simulink model "sysgenPatternGenerator"  (Simulink 7.1)
settings: Solver=VariableStepDiscrete  StartTime=0.0  StopTime=30000  RelTol=1e-3
PreLoadFcn:
  | load rgb;
  | fill_pattern_gen_program_store;
InitFcn:
  | load rgb;
  | fill_pattern_gen_program_store;
StopFcn:
  | makematrix(red, blue, green);
libraries: xbsIndex_r4 x47, xbsCopyrightNotice_r4 x1
settings Model: Creator=singhj  LastModifiedBy=sps
settings OptimizationCC: InlineInvariantSignals=on
settings DebuggingCC: SaveWithParameterizedLinksMsg=none  SignalResolutionControl=TryResolveAllWithWarning  SolverPrmCheckMsg=none  MultiTaskDSMMsg=warning  MultiTaskCondExecSysMsg=none  StrictBusMsg=None
settings RTWCC: IncludeERTFirstTime=on
settings GRTTargetCC: TargetFcnLib=ansi_tfl_tmw.mat

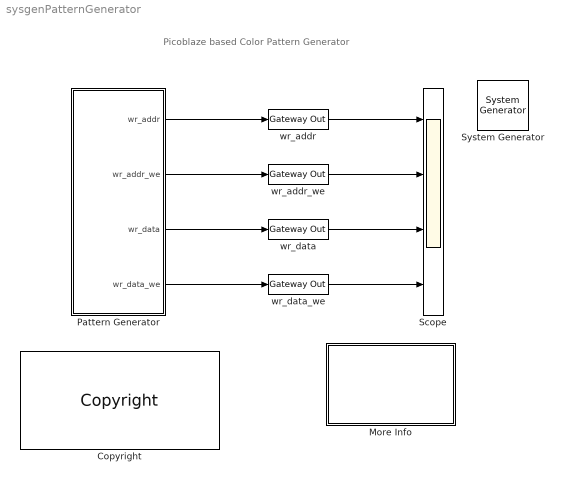
== system sysgenPatternGenerator ==
  note: Picoblaze based Color Pattern Generator
  " System Generator" : xbsIndex_r4/ System Generator  Tag=genX  SystemSampleTime=-1  xilinxfamily=virtex6  part=xc6vlx240t  speed=-1  package=ff1156  synthesis_tool=XST  clock_wrapper=Clock Enables  directory=./netlist  testbench=on  simulink_period=1  sysclk_period=10  dcm_input_clock_period=100  incr_netlist=off  trim_vbits=Everywhere in SubSystem  dbl_ovrd=According to Block Masks  core_generation=According to Block Masks  run_coregen=off  deprecated_control=off  eval_field=0  block_type=sysgen
      settings: block_version=9.2.00
  Copyright : xbsCopyrightNotice_r4/Copyright  copyrighttext="Copyright (c) 2010  by  Xilinx, Inc. All rights reserved.<br><br>This file contains proprietary, confidential information of Xilinx, Inc., is distributed under licensefrom Xilinx, Inc., and may be used, copied and/or disclosed only pursuant to the terms of a valid licenseagreement with Xilinx, Inc. Xilinx hereby grants you a license to use this file solely for design,simulation, implementation and creation of design files limited to Xilinx devices or technologies. Use with non-Xilinx devices or technologies is expressly prohibited and immediately terminates your license unless covered by a separate agreement.<br><br>Xilinx is providing this design, code, or information \"as-is\" solely for use in developing programs and solutions for Xilinx devices, with no obligation on the part of Xilinx to provide support. By providingthis design, code, or information as one possible implementation of this feature, application or standard,Xilinx is making no representation that this implementation is free from any claims of infringement. Youare responsible for obtaining any rights you may require for your implementation. Xilinx expressly disclaimsany warranty whatsoever with respect to the adequacy of the implementation, including but not limited to anywarranties or representations that this implementation is free from claims of infringement, implied warrantiesof merchantability or fitness for a particular purpose.<br><br>Xilinx products are not intended for use in life support appliances, devices, or systems. Use in such applications is expressly prohibited.<br><br>Any modifications that are made to the Source Code are done at the user's sole risk and will be unsupported.<br><br>This copyright and support notice must be retained as part of this text at all times. (c) Copyright 1995-2010 Xilinx, Inc. All rights reserved."  block_type=copyright
      settings: block_version=10.1.00
      settings: infoedit=|
      | Copyright(C) 2008 by  Xilinx, Inc. All rights reserved.<br>
      | <br>
      | This file contains proprietary, confidential information of Xilinx, Inc., is distributed under license
      | from Xilinx, Inc., and may be used, copied and/or disclosed only pursuant to the terms of a valid license
      | agreement with Xilinx, Inc. Xilinx hereby grants you a license to use this file solely for design,
      | simulation, implementation and creation of design files limited to Xilinx devices or technologies. Use
      | with non-Xilinx devices or technologies is expressly prohibited and immediately terminates your license
      | unless covered by a separate agreement.<br>
      | <br>
      | Xilinx is providing this design, code, or information "as-is" solely for use in developing programs and
      | solutions for Xilinx devices, with no obligation on the part of Xilinx to provide support. By providing
      | this design, code, or information as one possible implementation of this feature, application or standard,
      | Xilinx is making no representation that this implementation is free from any claims of infringement. You
      | are responsible for obtaining any rights you may require for your implementation. Xilinx expressly disclaims
      | any warranty whatsoever with respect to the adequacy of the implementation, including but not limited to any
      | warranties or representations that this implementation is free from claims of infringement, implied warranties
      | of merchantability or fitness for a particular purpose.<br>
      | <br>
      | Xilinx products are not intended for use in life support appliances, devices, or systems. Use in such
      | applications is expressly prohibited.<br>
      | <br>
      | Any modifications that are made to the Source Code are done at the user's sole risk and will be unsupported.<br>
      | <br>
      | This copyright and support notice must be retained as part of this text at all times.
      | (c) Copyright 1995-2008 Xilinx, Inc. All rights reserved.
  More Info : Subsystem
      mask Display: disp('Double click\n for\n more information.')
  Pattern Generator : Subsystem
  Scope : Scope  NumInputPorts=4
      settings: YMin=1.02005e+009~0~0~0  YMax=1.12743e+009~1~1.75e+007~1
  wr_addr : xbsIndex_r4/Gateway Out  hdl_port=on  timing_constraint=None  locs_specified=off  LOCs={}  block_type=gatewayout
      settings: infoedit="Gateway out block.  Converts Xilinx fixed point inputs into ouputs of type Simulink integer, double, or fixed point.<P><P>Hardware notes:  In hardware these blocks become top level output ports or are discarded, depending on how they are configured."  block_version=VER_STRING_GOES_HERE
  wr_addr_we : xbsIndex_r4/Gateway Out  hdl_port=on  timing_constraint=None  locs_specified=off  LOCs={}  block_type=gatewayout
      settings: infoedit="Gateway out block.  Converts Xilinx fixed point inputs into ouputs of type Simulink integer, double, or fixed point.<P><P>Hardware notes:  In hardware these blocks become top level output ports or are discarded, depending on how they are configured."  block_version=VER_STRING_GOES_HERE
  wr_data : xbsIndex_r4/Gateway Out  hdl_port=on  timing_constraint=None  locs_specified=off  LOCs={}  block_type=gatewayout
      settings: infoedit="Gateway out block.  Converts Xilinx fixed point inputs into ouputs of type Simulink integer, double, or fixed point.<P><P>Hardware notes:  In hardware these blocks become top level output ports or are discarded, depending on how they are configured."  block_version=VER_STRING_GOES_HERE
  wr_data_we : xbsIndex_r4/Gateway Out  hdl_port=on  timing_constraint=None  locs_specified=off  LOCs={}  block_type=gatewayout
      settings: infoedit="Gateway out block.  Converts Xilinx fixed point inputs into ouputs of type Simulink integer, double, or fixed point.<P><P>Hardware notes:  In hardware these blocks become top level output ports or are discarded, depending on how they are configured."  block_version=VER_STRING_GOES_HERE
  wires:
  wr_addr/1 -> Scope/1
  wr_data/1 -> Scope/3
  Pattern Generator/4(wr_data_we) -> wr_data_we/1
  wr_data_we/1 -> Scope/4
  Pattern Generator/1(wr_addr) -> wr_addr/1
  Pattern Generator/3(wr_data) -> wr_data/1
  wr_addr_we/1 -> Scope/2
  Pattern Generator/2(wr_addr_we) -> wr_addr_we/1

== system sysgenPatternGenerator/More Info ==
  note: Picoblaze based Color Pattern Generator
  note: This design shows how the PicoBlaze soft processor can be used to generate an image for video display.
      | This demo includes a function to display the image in a Matlab figure window.
      |
      | The pattern generator is intended to be connected to the UltraMC SDRAM memory controller (not included in
      |  this demo).  The four output ports on the "Pattern Generator" subsystem interface directly to a 32-bit write port
      | on the UltraMC.

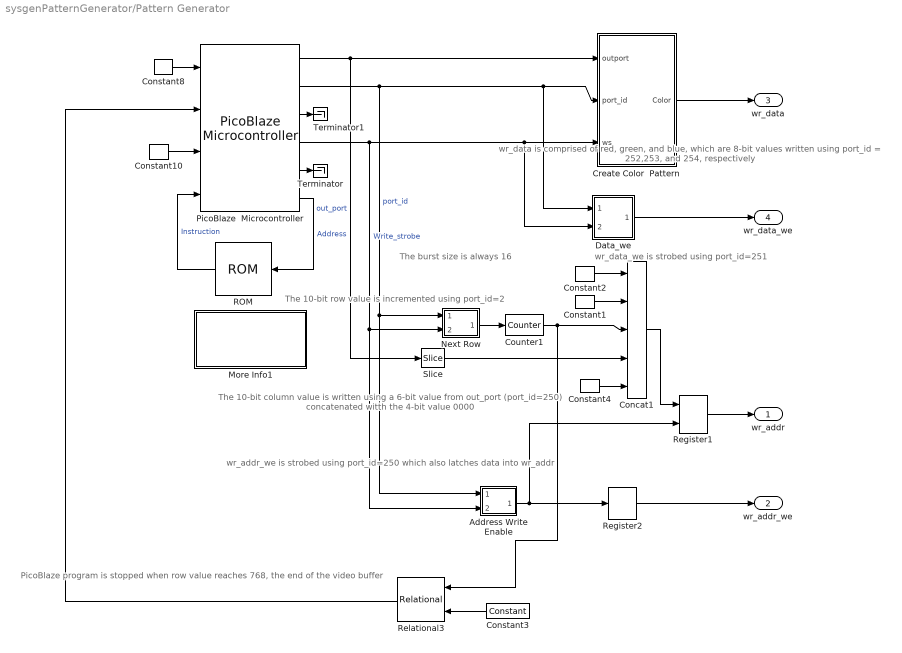
== system sysgenPatternGenerator/Pattern Generator ==
  note: The burst size is always 16
  note: The 10-bit row value is
      | incremented using port_id=2
  note: wr_data_we is strobed
      | using port_id=251
  note: wr_addr_we is strobed
      | using port_id=250 which also
      | latches data into wr_addr
  note: PicoBlaze program is stopped when
      | row value reaches 768, the end of the
      | video buffer
  note: wr_data is comprised of red,
      | green, and blue, which are
      | 8-bit values written using
      | port_id = 252,253, and 254,
      | respectively
  note: The 10-bit column value is
      | written using a 6-bit value from
      | out_port (port_id=250) concatenated
      | witth the 4-bit value 0000
  Address Write Enable : Subsystem
  Concat1 : xbsIndex_r4/Concat  num_inputs=5  dbl_ovrd=off  block_type=concat
      settings: block_version=VER_STRING_GOES_HERE
  Constant1 : xbsIndex_r4/Constant  arith_type=Unsigned  const=0  n_bits=6  bin_pt=0  explicit_period=off  period=1  equ=P=C  opselect=C  inp2=PCIN>>17  opr=+  inp1=P  carry=CIN  dbl_ovrd=off  block_type=constant
      settings: block_version=VER_STRING_GOES_HERE
  Constant10 : xbsIndex_r4/Constant  arith_type=Boolean  const=0  n_bits=8  bin_pt=0  explicit_period=on  period=eval(get_param([bdroot,'/ System Generator'],'simulink_period'));  equ=P=C  opselect=C  inp2=PCIN>>17  opr=+  inp1=P  carry=CIN  dbl_ovrd=off  block_type=constant
      settings: block_version=VER_STRING_GOES_HERE
  Constant2 : xbsIndex_r4/Constant  arith_type=Unsigned  const=16  n_bits=10  bin_pt=0  explicit_period=off  period=1  equ=P=C  opselect=C  inp2=PCIN>>17  opr=+  inp1=P  carry=CIN  dbl_ovrd=off  block_type=constant
      settings: block_version=VER_STRING_GOES_HERE
  Constant3 : xbsIndex_r4/Constant  arith_type=Unsigned  const=768  n_bits=10  bin_pt=0  explicit_period=off  period=1  equ=P=C  opselect=C  inp2=PCIN>>17  opr=+  inp1=P  carry=CIN  dbl_ovrd=off  block_type=constant
      settings: block_version=VER_STRING_GOES_HERE
  Constant4 : xbsIndex_r4/Constant  arith_type=Unsigned  const=0  n_bits=4  bin_pt=0  explicit_period=off  period=1  equ=P=C  opselect=C  inp2=PCIN>>17  opr=+  inp1=P  carry=CIN  dbl_ovrd=off  block_type=constant
      settings: block_version=VER_STRING_GOES_HERE
  Constant8 : xbsIndex_r4/Constant  arith_type=Unsigned  const=0  n_bits=8  bin_pt=0  explicit_period=on  period=eval(get_param([bdroot,'/ System Generator'],'simulink_period'));  equ=P=C  opselect=C  inp2=PCIN>>17  opr=+  inp1=P  carry=CIN  dbl_ovrd=off  block_type=constant
      settings: block_version=VER_STRING_GOES_HERE
  Counter1 : xbsIndex_r4/Counter  cnt_type=Count Limited  cnt_to=767  operation=Up  start_count=0  cnt_by_val=1  arith_type=Unsigned  n_bits=10  bin_pt=0  load_pin=off  rst=off  en=on  explicit_period=on  period=eval(get_param([bdroot,'/ System Generator'],'simulink_period'));  dbl_ovrd=off  use_behavioral_HDL=off  implementation=Fabric  use_rpm=off  block_type=counter
      settings: block_version=VER_STRING_GOES_HERE
  Create Color  Pattern : Subsystem
  Data_we : Subsystem
  More Info1 : Subsystem
      settings: OpenFcn=edit('pattern_gen.psm')
      mask Display: disp('Double click to view\n  the Picoblaze \n  Assembly Code.')
  "Next Row " : Subsystem
  PicoBlaze  Microcontroller : xbsIndex_r4/PicoBlaze Microcontroller  version=PicoBlaze 3  display_mi=off  xl_view_as=Hexadecimal  block_type=pb
      settings: block_version=VER_STRING_GOES_HERE
  ROM : xbsIndex_r4/ROM  depth=1024  initVector=fill_pattern_gen_program_store  distributed_mem=Block RAM  rst=off  init_reg=0  en=off  latency=1  arith_type=Unsigned  n_bits=18  bin_pt=0  dbl_ovrd=off  optimize=Area  use_rpm=on  block_type=sprom
      settings: block_version=VER_STRING_GOES_HERE
  Register1 : xbsIndex_r4/Register  init=0  rst=off  en=on  dbl_ovrd=off  block_type=register
      settings: block_version=VER_STRING_GOES_HERE
  Register2 : xbsIndex_r4/Register  init=0  rst=off  en=off  dbl_ovrd=off  block_type=register
      settings: block_version=VER_STRING_GOES_HERE
  Relational3 : xbsIndex_r4/Relational  mode=a=b  en=off  latency=1  dbl_ovrd=off  block_type=relational
      settings: block_version=VER_STRING_GOES_HERE
  Slice : xbsIndex_r4/Slice  nbits=6  boolean_output=off  mode=Lower Bit Location + Width  bit1=0  base1=MSB of Input  bit0=0  base0=LSB of Input  dbl_ovrd=off  block_type=slice
      settings: infoedit="Extracts a given range of bits from each input sample and presents it at the output.  The output type is ordinarily unsigned with binary point at zero, but can be Boolean when the slice is one bit wide.<P><P>Hardware notes: In hardware this block costs nothing."  block_version=VER_STRING_GOES_HERE
  Terminator : Terminator
  Terminator1 : Terminator
  wr_addr : Outport  OutDataType=sfix(16)  OutScaling=2^0
  wr_addr_we : Outport  Port=2  OutDataType=sfix(16)  OutScaling=2^0
  wr_data : Outport  Port=3  OutDataType=sfix(16)  OutScaling=2^0
  wr_data_we : Outport  Port=4  OutDataType=sfix(16)  OutScaling=2^0
  wires:
  Concat1/1 -> Register1/1
  Constant4/1 -> Concat1/5
  Constant2/1 -> Concat1/1
  Constant1/1 -> Concat1/2
  Counter1/1 -> Relational3/1, Concat1/3
  "Next Row "/1(Out1) -> Counter1/1
  PicoBlaze  Microcontroller/4 -> Data_we/2(In2), Create Color  Pattern/3(ws), "Next Row "/2(In2), Address Write Enable/2(In2)  "Write_strobe"
  PicoBlaze  Microcontroller/1 -> Create Color  Pattern/1(outport), Slice/1  "out_port"
  PicoBlaze  Microcontroller/2 -> "Next Row "/1(In1), Address Write Enable/1(In1), Data_we/1(In1), Create Color  Pattern/2(port_id)  "port_id"
  PicoBlaze  Microcontroller/3 -> Terminator1/1
  PicoBlaze  Microcontroller/5 -> Terminator/1
  ROM/1 -> PicoBlaze  Microcontroller/4  "Instruction"
  PicoBlaze  Microcontroller/6 -> ROM/1  "Address"
  Constant8/1 -> PicoBlaze  Microcontroller/1
  Constant3/1 -> Relational3/2
  Relational3/1 -> PicoBlaze  Microcontroller/2
  Constant10/1 -> PicoBlaze  Microcontroller/3
  Register1/1 -> wr_addr/1
  Register2/1 -> wr_addr_we/1
  Create Color  Pattern/1(Color) -> wr_data/1
  Data_we/1(Out1) -> wr_data_we/1
  Slice/1 -> Concat1/4
  Address Write Enable/1(Out1) -> Register2/1, Register1/2

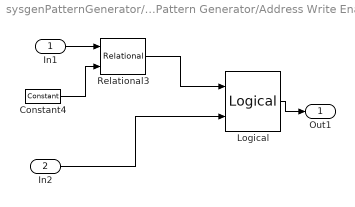
== system sysgenPatternGenerator/Pattern Generator/Address Write Enable ==
  In1 : Inport  OutDataType=sfix(16)  OutScaling=2^0
  In2 : Inport  Port=2  OutDataType=sfix(16)  OutScaling=2^0
  Constant4 : xbsIndex_r4/Constant  arith_type=Unsigned  const=250  n_bits=8  bin_pt=0  explicit_period=off  period=1  equ=P=C  opselect=C  inp2=PCIN>>17  opr=+  inp1=P  carry=CIN  dbl_ovrd=off  block_type=constant
      settings: block_version=VER_STRING_GOES_HERE
  Logical : xbsIndex_r4/Logical  logical_function=AND  inputs=2  en=off  latency=0  precision=Full  arith_type=Unsigned  n_bits=16  bin_pt=0  align_bp=on  dbl_ovrd=off  block_type=logical
      settings: block_version=VER_STRING_GOES_HERE
  Relational3 : xbsIndex_r4/Relational  mode=a=b  en=off  latency=1  dbl_ovrd=off  block_type=relational
      settings: block_version=VER_STRING_GOES_HERE
  Out1 : Outport  OutDataType=sfix(16)  OutScaling=2^0
  wires:
  In2/1 -> Logical/2
  Relational3/1 -> Logical/1
  Logical/1 -> Out1/1
  In1/1 -> Relational3/1
  Constant4/1 -> Relational3/2

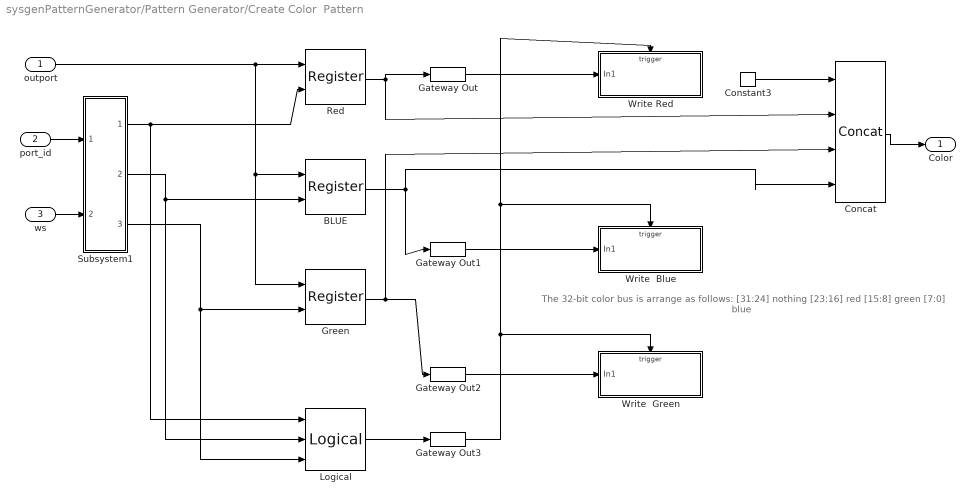
== system sysgenPatternGenerator/Pattern Generator/Create Color  Pattern ==
  note: The 32-bit color bus is arrange as follows:
      | [31:24] nothing
      | [23:16] red
      | [15:8] green
      | [7:0] blue
  outport : Inport  OutDataType=sfix(16)  OutScaling=2^0
  port_id : Inport  Port=2  OutDataType=sfix(16)  OutScaling=2^0
  ws : Inport  Port=3  OutDataType=sfix(16)  OutScaling=2^0
  BLUE : xbsIndex_r4/Register  init=0  rst=off  en=on  dbl_ovrd=off  block_type=register
      settings: block_version=VER_STRING_GOES_HERE
  Concat : xbsIndex_r4/Concat  num_inputs=4  dbl_ovrd=off  block_type=concat
      settings: block_version=VER_STRING_GOES_HERE
  Constant3 : xbsIndex_r4/Constant  arith_type=Unsigned  const=0  n_bits=8  bin_pt=0  explicit_period=off  period=1  equ=P=C  opselect=C  inp2=PCIN>>17  opr=+  inp1=P  carry=CIN  dbl_ovrd=off  block_type=constant
      settings: block_version=VER_STRING_GOES_HERE
  Gateway Out{,1..3} (4 alike) : xbsIndex_r4/Gateway Out  hdl_port=off  timing_constraint=None  locs_specified=off  LOCs={}  block_type=gatewayout
      settings: infoedit="Gateway out block.  Converts Xilinx fixed point inputs into ouputs of type Simulink integer, double, or fixed point.<br><br>Hardware notes:  In hardware these blocks become top level output ports or are discarded, depending on how they are configured."  block_version=11.3
  Green : xbsIndex_r4/Register  init=0  rst=off  en=on  dbl_ovrd=off  block_type=register
      settings: block_version=VER_STRING_GOES_HERE
  Logical : xbsIndex_r4/Logical  logical_function=OR  inputs=3  en=off  latency=0  precision=Full  arith_type=Unsigned  n_bits=16  bin_pt=0  align_bp=on  dbl_ovrd=off  block_type=logical
      settings: block_version=VER_STRING_GOES_HERE
  Red : xbsIndex_r4/Register  init=0  rst=off  en=on  dbl_ovrd=off  block_type=register
      settings: block_version=VER_STRING_GOES_HERE
  Subsystem1 : Subsystem
  Write Red : Subsystem  TreatAsAtomicUnit=on
  Write  Blue : Subsystem  TreatAsAtomicUnit=on
  Write  Green : Subsystem  TreatAsAtomicUnit=on
  Color : Outport  OutDataType=sfix(16)  OutScaling=2^0
  wires:
  ws/1 -> Subsystem1/2(In2)
  port_id/1 -> Subsystem1/1(In1)
  outport/1 -> Red/1, Green/1, BLUE/1
  Red/1 -> Gateway Out/1, Concat/2
  Subsystem1/3(green en) -> Green/2, Logical/3
  Subsystem1/2(blue en) -> Logical/2, BLUE/2
  BLUE/1 -> Gateway Out1/1, Concat/4
  Green/1 -> Gateway Out2/1, Concat/3
  Constant3/1 -> Concat/1
  Subsystem1/1(red en) -> Logical/1, Red/2
  Concat/1 -> Color/1
  Logical/1 -> Gateway Out3/1
  Gateway Out/1 -> Write Red/1(In1)
  Gateway Out1/1 -> Write  Blue/1(In1)
  Gateway Out2/1 -> Write  Green/1(In1)
  Gateway Out3/1 -> Write Red/Trigger, Write  Blue/Trigger, Write  Green/Trigger

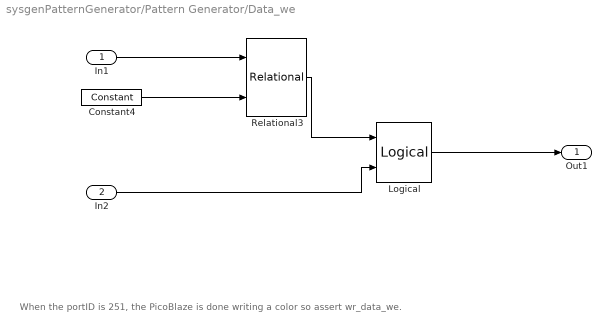
== system sysgenPatternGenerator/Pattern Generator/Data_we ==
  note: When the portID is 251, the PicoBlaze is done writing a color so assert wr_data_we.
  In1 : Inport  OutDataType=sfix(16)  OutScaling=2^0
  In2 : Inport  Port=2  OutDataType=sfix(16)  OutScaling=2^0
  Constant4 : xbsIndex_r4/Constant  arith_type=Unsigned  const=251  n_bits=8  bin_pt=0  explicit_period=off  period=1  equ=P=C  opselect=C  inp2=PCIN>>17  opr=+  inp1=P  carry=CIN  dbl_ovrd=off  block_type=constant
      settings: block_version=VER_STRING_GOES_HERE
  Logical : xbsIndex_r4/Logical  logical_function=AND  inputs=2  en=off  latency=0  precision=Full  arith_type=Unsigned  n_bits=16  bin_pt=0  align_bp=on  dbl_ovrd=off  block_type=logical
      settings: block_version=VER_STRING_GOES_HERE
  Relational3 : xbsIndex_r4/Relational  mode=a=b  en=off  latency=1  dbl_ovrd=off  block_type=relational
      settings: block_version=VER_STRING_GOES_HERE
  Out1 : Outport  OutDataType=sfix(16)  OutScaling=2^0
  wires:
  Logical/1 -> Out1/1
  In2/1 -> Logical/2
  Relational3/1 -> Logical/1
  In1/1 -> Relational3/1
  Constant4/1 -> Relational3/2

== system sysgenPatternGenerator/Pattern Generator/More Info1 ==

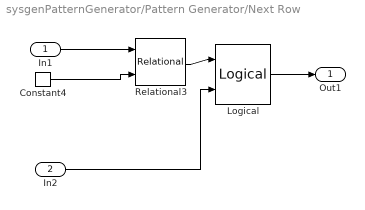
== system sysgenPatternGenerator/Pattern Generator/Next Row  ==
  In1 : Inport  OutDataType=sfix(16)  OutScaling=2^0
  In2 : Inport  Port=2  OutDataType=sfix(16)  OutScaling=2^0
  Constant4 : xbsIndex_r4/Constant  arith_type=Unsigned  const=2  n_bits=8  bin_pt=0  explicit_period=off  period=1  equ=P=C  opselect=C  inp2=PCIN>>17  opr=+  inp1=P  carry=CIN  dbl_ovrd=off  block_type=constant
      settings: block_version=VER_STRING_GOES_HERE
  Logical : xbsIndex_r4/Logical  logical_function=AND  inputs=2  en=off  latency=0  precision=Full  arith_type=Unsigned  n_bits=16  bin_pt=0  align_bp=on  dbl_ovrd=off  block_type=logical
      settings: block_version=VER_STRING_GOES_HERE
  Relational3 : xbsIndex_r4/Relational  mode=a=b  en=off  latency=1  dbl_ovrd=off  block_type=relational
      settings: block_version=VER_STRING_GOES_HERE
  Out1 : Outport  OutDataType=sfix(16)  OutScaling=2^0
  wires:
  Relational3/1 -> Logical/1
  In2/1 -> Logical/2
  Logical/1 -> Out1/1
  In1/1 -> Relational3/1
  Constant4/1 -> Relational3/2

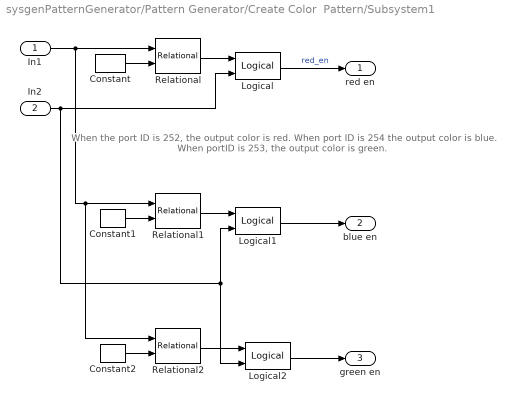
== system sysgenPatternGenerator/Pattern Generator/Create Color  Pattern/Subsystem1 ==
  note: When the port ID is 252, the output
      | color is red.  When port ID is 254 the
      | output color is blue.  When portID is
      | 253, the output color is green.
  In1 : Inport  OutDataType=sfix(16)  OutScaling=2^0
  In2 : Inport  Port=2  OutDataType=sfix(16)  OutScaling=2^0
  Constant : xbsIndex_r4/Constant  arith_type=Unsigned  const=252  n_bits=8  bin_pt=0  explicit_period=off  period=1  equ=P=C  opselect=C  inp2=PCIN>>17  opr=+  inp1=P  carry=CIN  dbl_ovrd=off  block_type=constant
      settings: block_version=VER_STRING_GOES_HERE
  Constant1 : xbsIndex_r4/Constant  arith_type=Unsigned  const=254  n_bits=8  bin_pt=0  explicit_period=off  period=1  equ=P=C  opselect=C  inp2=PCIN>>17  opr=+  inp1=P  carry=CIN  dbl_ovrd=off  block_type=constant
      settings: block_version=VER_STRING_GOES_HERE
  Constant2 : xbsIndex_r4/Constant  arith_type=Unsigned  const=253  n_bits=8  bin_pt=0  explicit_period=off  period=1  equ=P=C  opselect=C  inp2=PCIN>>17  opr=+  inp1=P  carry=CIN  dbl_ovrd=off  block_type=constant
      settings: block_version=VER_STRING_GOES_HERE
  Logical : xbsIndex_r4/Logical  logical_function=AND  inputs=2  en=off  latency=0  precision=Full  arith_type=Unsigned  n_bits=16  bin_pt=0  align_bp=on  dbl_ovrd=off  block_type=logical
      settings: block_version=VER_STRING_GOES_HERE
  Logical1 : xbsIndex_r4/Logical  logical_function=AND  inputs=2  en=off  latency=0  precision=Full  arith_type=Unsigned  n_bits=16  bin_pt=0  align_bp=on  dbl_ovrd=off  block_type=logical
      settings: block_version=VER_STRING_GOES_HERE
  Logical2 : xbsIndex_r4/Logical  logical_function=AND  inputs=2  en=off  latency=0  precision=Full  arith_type=Unsigned  n_bits=16  bin_pt=0  align_bp=on  dbl_ovrd=off  block_type=logical
      settings: block_version=VER_STRING_GOES_HERE
  Relational : xbsIndex_r4/Relational  mode=a=b  en=off  latency=1  dbl_ovrd=off  block_type=relational
      settings: block_version=VER_STRING_GOES_HERE
  Relational1 : xbsIndex_r4/Relational  mode=a=b  en=off  latency=1  dbl_ovrd=off  block_type=relational
      settings: block_version=VER_STRING_GOES_HERE
  Relational2 : xbsIndex_r4/Relational  mode=a=b  en=off  latency=1  dbl_ovrd=off  block_type=relational
      settings: block_version=VER_STRING_GOES_HERE
  red en : Outport  OutDataType=sfix(16)  OutScaling=2^0
  blue en : Outport  Port=2  OutDataType=sfix(16)  OutScaling=2^0
  green en : Outport  Port=3  OutDataType=sfix(16)  OutScaling=2^0
  wires:
  Logical2/1 -> green en/1
  Relational2/1 -> Logical2/1
  Logical1/1 -> blue en/1
  Relational1/1 -> Logical1/1
  Relational/1 -> Logical/1
  Logical/1 -> red en/1  "red_en"
  In2/1 -> Logical2/2, Logical1/2, Logical/2
  In1/1 -> Relational2/1, Relational1/1, Relational/1
  Constant2/1 -> Relational2/2
  Constant1/1 -> Relational1/2
  Constant/1 -> Relational/2

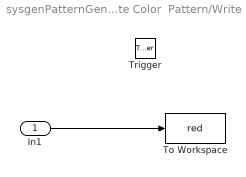
== system sysgenPatternGenerator/Pattern Generator/Create Color  Pattern/Write Red ==
  In1 : Inport  OutDataType=sfix(16)  OutScaling=2^0
  Trigger : TriggerPort
  To Workspace : ToWorkspace  VariableName=red  SampleTime=-1  SaveFormat=Array
      settings: MaxDataPoints=256
  wires:
  In1/1 -> To Workspace/1

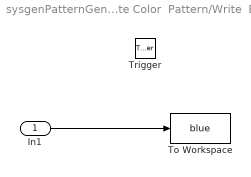
== system sysgenPatternGenerator/Pattern Generator/Create Color  Pattern/Write  Blue ==
  In1 : Inport  OutDataType=sfix(16)  OutScaling=2^0
  Trigger : TriggerPort
  To Workspace : ToWorkspace  VariableName=blue  SampleTime=-1  SaveFormat=Array
      settings: MaxDataPoints=256
  wires:
  In1/1 -> To Workspace/1

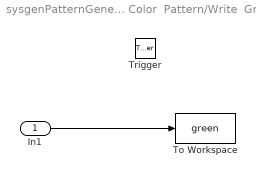
== system sysgenPatternGenerator/Pattern Generator/Create Color  Pattern/Write  Green ==
  In1 : Inport  OutDataType=sfix(16)  OutScaling=2^0
  Trigger : TriggerPort
  To Workspace : ToWorkspace  VariableName=green  SampleTime=-1  SaveFormat=Array
      settings: MaxDataPoints=256
  wires:
  In1/1 -> To Workspace/1
